simulink model "s32ze_counter_pil_simulink_r52"  (R2024b)
settings: Solver=FixedStepDiscrete  StartTime=0.0  StopTime=10.0  FixedStep=Auto  RelTol=1e-3  EnableMultiTasking=on
PreLoadFcn:
  | % NXP_MBDT_S32ZE callback: DO NOT REMOVE
  | mbd_s32ze.common.nxp.model_callbacks.preLoadFcn();
PostLoadFcn:
  | Increment = Simulink.Parameter;
  | Increment.DataType = 'uint8';
  | Increment.CoderInfo.StorageClass = 'SimulinkGlobal';
  | Increment.Value = 1;
  | 
  | SilCounterBus = Simulink.Bus;
  | SilCounterBus.Description = 'This bus contains counter inputs';
  | 
  | e1 = Simulink.BusElement;
  | e1.DataType = 'boolean';
  | e1.Name = 'ticks_to_count';
  | 
  | e2 = Simulink.BusElement;
  | e2.DataType = 'boolean';
  | e2.Name = 'reset';
  | 
  | SilCounterBus.Elements = [e1 e2];
  | clear e1 e2
  | 
  | % Step size
  | T=0.1;
  | 
  | % Input values
  | ticks_to_count.time = (0:100)'*T;
  | ticks_to_count.signals.values = boolean((floor( (0:100)/2)==(0:100)/2)');
  | ticks_to_count.signals.dimensions = 1;
  | 
  | reset.time = (0:100)'*T;
  | reset_values = boolean(zeros(101,1)); reset_values(20)=true;
  | reset.signals.values = reset_values;
  | clear reset_values
  | reset.signals.dimensions = 1;
  | % NXP_MBDT_S32ZE callback: DO NOT REMOVE
  | mbd_s32ze.common.nxp.model_callbacks.postLoadFcn();
InitFcn:
  | % NXP_MBDT_S32ZE callback: DO NOT REMOVE
  | mbd_s32ze.common.nxp.model_callbacks.initFcn();
model workspace (MATLAB code in the model file):
  | myLower = Simulink.Parameter;
  | myLower.Value = uint8(0);
  | 
  | myUpper = Simulink.Parameter;
  | myUpper.Value = uint8(10);
Description:
  | Example model reference component.
settings Model: DataDictionary=s32ze_counter_pil_simulink_r52.sldd  ParameterArgumentNames=myLower,myUpper  Creator=The MathWorks, Inc.  LastModifiedBy=nxg00842
settings SolverCC: AlgebraicLoopSolver=TrustRegion
settings DataIOCC: SaveFormat=StructureWithTime  SaveOutput=off  SaveTime=off  ReturnWorkspaceOutputs=off  SignalLoggingName=logsOut
settings OptimizationCC: UseDivisionForNetSlopeComputation=UseDivisionForReciprocalsOfIntegersOnly  EnhancedBackFolding=on  BooleansAsBitfields=on  PassReuseOutputArgsAs=Individual arguments  ExpressionDepthLimit=2147483647  StateBitsets=on  DataBitsets=on  ZeroExternalMemoryAtStartup=off  ZeroInternalMemoryAtStartup=off  NoFixptDivByZeroProtection=on  EfficientFloat2IntCast=on  LifeSpan=1  MaxStackSize=64  SimCompilerOptimization=on  EfficientTunableParamExpr=on
settings DebuggingCC: ReadBeforeWriteMsg=DisableAll  WriteAfterWriteMsg=DisableAll  WriteAfterReadMsg=DisableAll  UnderspecifiedInitializationDetection=Classic  CheckExecutionContextPreStartOutputMsg=on  InheritedTsInSrcMsg=none  FcnCallInpInsideContextMsg=warning  UnconnectedInputMsg=warning  UnconnectedOutputMsg=warning  UnconnectedLineMsg=warning  UniqueDataStoreMsg=error  AllowSymbolicDim=off  ModelReferenceSymbolNameMessage=none  StateNameClashWarn=warning  StrictBusMsg=ErrorOnBusTreatedAsVector  SFUnexpectedBacktrackingDiag=warning  SFNoUnconditionalDefaultTransitionDiag=warning  SFExecutionAtInitializationDiag=none  ArithmeticOperatorsInVariantConditions=warning
settings HardwareCC: ProdBitPerPointer=32  ProdBitPerSizeT=32  ProdBitPerPtrDiffT=32  ProdLargestAtomicInteger=Long  ProdLargestAtomicFloat=Double  ProdWordSize=32  ProdHWDeviceType=ARM Compatible->ARM Cortex  TargetHWDeviceType=Generic->32-bit Embedded Processor
settings ModelReferenceCC: EnableRefExpFcnMdlSchedulingChecks=on  CheckModelReferenceTargetMessage=none  ModelReferencePassRootInputsByReference=off  PropagateSignalLabelsOutOfModel=off
settings SFSimCC: SimUseLocalCustomCode=off  MATLABDynamicMemAlloc=off  CustomCodeUndefinedFunction=UseInterfaceOnly
settings RTWCC: Description=Embedded Coder  SystemTargetFile=ert.tlc  HardwareBoard=NXP S32ZE2xx  TemplateMakefile=ert_default_tmf  GenerateReport=on  RTWVerbose=off  RTWUseLocalCustomCode=off  Toolchain=NXP S32 Design Studio GCC (S32ZE)  BuildConfiguration=Faster Runs  IncludeHyperlinkInReport=on  CodeExecutionProfiling=on  CodeProfilingInstrumentation=coarse  GenerateTraceInfo=on  GenerateTraceReport=on  GenerateTraceReportSl=on  GenerateTraceReportSf=on  GenerateTraceReportEml=on  GPUComputeCapability=3.5  DLArmComputeVersion=19.05
settings CodeAppCC: ForceParamTrailComments=on  IgnoreCustomStorageClasses=off  SimulinkDataObjDesc=on  CustomSymbolStrGlobalVar=rt$N$M  CustomSymbolStrType=$N$M  CustomSymbolStrFcn=$N$M$F  CustomSymbolStrMacro=$N$M  InsertBlockDesc=on  StateflowObjectComments=on  InternalIdentifier=Classic
settings ERTTargetCC: UtilityFuncGeneration=Shared location  MultiwordLength=2048  IncludeMdlTerminateFcn=off  CombineSignalStateStructs=on  SupportAbsoluteTime=off  SupportNonFinite=off  SupportComplex=off  SupportNonInlinedSFcns=on  ExtModeTransport=1  ExtModeMexFile=ext_serial_win32_comm  InlinedParameterPlacement=Hierarchical  ERTSrcFileBannerTemplate=mbd_s32ze_ert_code_template.cgt  ERTHdrFileBannerTemplate=mbd_s32ze_ert_code_template.cgt  ERTDataSrcFileTemplate=mbd_s32ze_ert_code_template.cgt  ERTDataHdrFileTemplate=mbd_s32ze_ert_code_template.cgt  ERTFilePackagingFormat=CompactWithDataFile  ConvertIfToSwitch=off  SuppressUnreachableDefaultCases=off  DynamicArrayContainerType=coder::array
settings ConfigComp: CovMetricSettings=dw  CovSaveCumulativeToWorkspaceVar=on  CovSaveSingleToWorkspaceVar=on  CovExternalEMLEnable=off  CovSFcnEnable=off

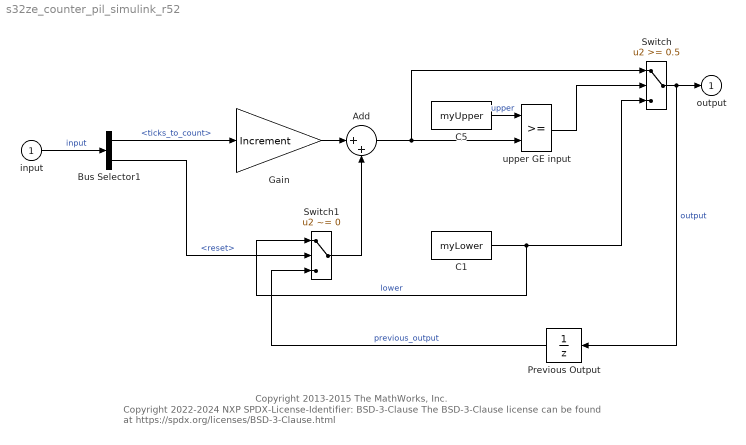
== system s32ze_counter_pil_simulink_r52 ==
  note: Copyright 2013-2015 The MathWorks, Inc.
  note: Copyright 2022-2024 NXP
      |
      | SPDX-License-Identifier: BSD-3-Clause
      | The BSD-3-Clause license can be found at https://spdx.org/licenses/BSD-3-Clause.html
  " input" : Inport  OutDataTypeStr=Bus: SilCounterBus  PortDimensions=1
  Add : Sum  Inputs=|++
  Bus Selector1 : BusSelector  OutputSignals=ticks_to_count,reset
  C1 : Constant  Value=myLower  OutDataTypeStr=uint8
  C5 : Constant  Value=myUpper  OutDataTypeStr=uint8
  Gain : Gain  Gain=Increment  ParamDataTypeStr=uint8  OutDataTypeStr=uint8
  Previous Output : UnitDelay  InitialCondition=50  SampleTime=-1  HasFrameUpgradeWarning=on
  Switch : Switch  Threshold=0.5  SaturateOnIntegerOverflow=off
  Switch1 : Switch  Criteria=u2 ~= 0  Threshold=0.5  SaturateOnIntegerOverflow=off
  upper GE input : RelationalOperator  Priority=0
      settings: AttributesFormatString=\n
  output : Outport  VectorParamsAs1DForOutWhenUnconnected=off
  wires:
  Switch/1 -> output/1, Previous Output/1  "output"
  upper GE input/1 -> Switch/2
  " input"/1 -> Bus Selector1/1  "input"
  C5/1 -> upper GE input/1  "upper"
  Add/1 -> upper GE input/2, Switch/1
  Gain/1 -> Add/1
  C1/1 -> Switch/3, Switch1/1  "lower"
  Bus Selector1/1 -> Gain/1  "<ticks_to_count>"
  Bus Selector1/2 -> Switch1/2  "<reset>"
  Previous Output/1 -> Switch1/3  "previous_output"
  Switch1/1 -> Add/2
